simulink model "trigger"  (R2013a)
settings: Solver=VariableStepDiscrete  StartTime=0.0  StopTime=1500  RelTol=1e-3
InitFcn:
  | fs=3e3;
  | lpfB=[0.000321846973661, 0.000573337526427, 0.001013809349453, 0.001105752673372, 0.001013809349453, 0.000573337526427, 0.000321846973661];
  | lpfA=[1.000000000000000, -4.802276968769980, 10.285791458772811, -12.473473099846858, 9.002976469782535, -3.665002072820574, 0.658939181018130];
  | windowSize=1000;
  | alpha=2e-6;
libraries: simulink x1
settings Model: Creator=balazs.varga  LastModifiedBy=balazs.varga

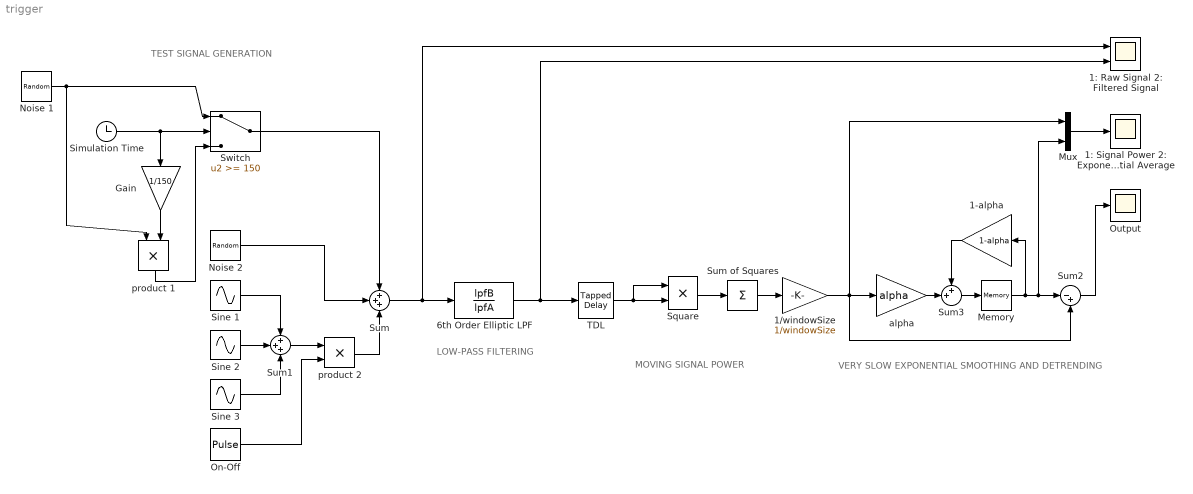
== system trigger ==
  note: VERY SLOW EXPONENTIAL SMOOTHING
      | AND DETRENDING
  note: MOVING SIGNAL POWER
  note: TEST SIGNAL GENERATION
  note: LOW-PASS FILTERING
  1-alpha : Gain  Gain=1-alpha  SampleTime=1/fs
  1/windowSize : Gain  Gain=1/windowSize  SampleTime=1/fs
  1: Raw Signal 2: Filtered Signal : Scope  NumInputPorts=2
      settings: YMin=-5~-5  YMax=5~5
  1: Signal Power 2: Exponential Average : Scope
      settings: YMin=0  YMax=525  SaveName=ScopeData3
  6th Order Elliptic LPF : DiscreteFilter  Numerator=lpfB  Denominator=lpfA  SampleTime=1/fs
  Gain : Gain  Gain=1/150  SampleTime=1/fs
  Memory : Memory  InheritSampleTime=on
  Mux : Mux  Inputs=2
  Noise 1 : RandomNumber  Variance=0.3  SampleTime=1/fs
  Noise 2 : RandomNumber  Variance=0.3  SampleTime=1/fs
  On-Off : DiscretePulseGenerator  PulseType=Time based  Period=100  PulseWidth=10  PhaseDelay=-12
  Output : Scope
      settings: YMin=-0.06  YMax=0.04  SaveName=ScopeData2
  Simulation Time : Clock
  Sine 1 : Sin  Amplitude=0  Frequency=2*pi*101  SampleTime=0
  Sine 2 : Sin  Amplitude=0  Frequency=2*pi*190  SampleTime=0
  Sine 3 : Sin  Frequency=2*pi*312  SampleTime=0
  Square : Product  SampleTime=1/fs
  Sum : Sum  Inputs=+++  SampleTime=1/fs
  Sum of Squares : Sum  Inputs=+  SampleTime=1/fs
  Sum1 : Sum  Inputs=+++  SampleTime=1/fs
  Sum2 : Sum  Inputs=|-+  SampleTime=1/fs
  Sum3 : Sum  Inputs=++|  SampleTime=1/fs
  Switch : Switch  Threshold=150  SampleTime=1/fs
  TDL : simulink/Discrete/Tapped Delay  vinit=0.0  samptime=1/fs  NumDelays=windowSize-1  DelayOrder=Newest  includeCurrent=on
  alpha : Gain  Gain=alpha  SampleTime=1/fs
  product 1 : Product  SampleTime=1/fs
  product 2 : Product  SampleTime=1/fs
  wires:
  On-Off/1 -> product 2/2
  Sum/1 -> 6th Order Elliptic LPF/1, 1: Raw Signal 2: Filtered Signal/1
  Sine 2/1 -> Sum1/2
  Sine 1/1 -> Sum1/1
  Sine 3/1 -> Sum1/3
  Sum1/1 -> product 2/1
  6th Order Elliptic LPF/1 -> 1: Raw Signal 2: Filtered Signal/2, TDL/1
  TDL/1 -> Square/2, Square/1
  Square/1 -> Sum of Squares/1
  Simulation Time/1 -> Gain/1, Switch/2
  Noise 1/1 -> product 1/1, Switch/1
  Switch/1 -> Sum/1
  product 2/1 -> Sum/3
  Noise 2/1 -> Sum/2
  product 1/1 -> Switch/3
  Gain/1 -> product 1/2
  Sum3/1 -> Memory/1
  alpha/1 -> Sum3/2
  1-alpha/1 -> Sum3/1
  Memory/1 -> 1-alpha/1, Sum2/1, Mux/2
  Mux/1 -> 1: Signal Power 2: Exponential Average/1
  Sum of Squares/1 -> 1/windowSize/1
  Sum2/1 -> Output/1
  1/windowSize/1 -> alpha/1, Sum2/2, Mux/1
